simulink model "ZSM_TeslaModelS_statKreisfahrt"  (R2020b)
settings: Solver=FixedStepDiscrete  StartTime=0.0  StopTime=simtime  FixedStep=stepsize  RelTol=1e-3
undefined symbols (not defined in the file): activate_stop, activate_stop_vmax, ay_stop, ayObs, ayStiff, Bat_param, deltav_ist, DiscIntNeverNeededParam, EG_wunsch, magnitude, mu_road_LF, mu_road_LR, mu_road_RF, mu_road_RR, par_ASR, par_MDT, par_TIR, par_VEH, select_delta_h, select_M_wheel, stepsize, t, temp_betriebsstrategie, temperature_LTrange, track_left, track_right
libraries: Library_ASK x36, simulink x16, pid_lib x2, dspstat3 x2, Library_Betriebsstrategie x2, vehicle_model x2, pacejka_trans x1
(part 7 of 7)

== matlab function ZSM_TeslaModelS_statKreisfahrt/Vehicle/Betriebsstrategie/Momentenverteilung_und_Schaltstrategie1/Radmomentenaufteilung (Standardfahrmanöver)/Schaltstrategie/Schaltlogik ==
  data: delta_n_LF input; delta_n_RF input; delta_n_LR input; delta_n_RR input; delta_n_F input; delta_n_R input; delta_m_LF input; delta_m_RF input; delta_m_LR input; delta_m_RR input; delta_m_F input; delta_m_R input; idx_LF_eff input; idx_RF_eff input; idx_LR_eff input; idx_RR_eff input; idx_F_eff input; idx_R_eff input; i_LF output; i_RF output; i_LR output; i_RR output; i_F output; iv_LF input; iv_RF input; iv_LR input; iv_RR input; iv_F input; iv_R input; i_R output; idx_LF output; idx_RF output; idx_LR output; idx_RR output; idx_F output; idx_R output; idx_LF_alt input; idx_RF_alt input; idx_LR_alt input; idx_RR_alt input; idx_F_alt input; idx_R_alt input
function [i_LF, i_RF, i_LR, i_RR, i_F, i_R, idx_LF, idx_RF, idx_LR, idx_RR, idx_F, idx_R] = fcn(delta_n_LF, delta_n_RF, delta_n_LR, delta_n_RR, delta_n_F, delta_n_R, delta_m_LF, delta_m_RF, delta_m_LR, delta_m_RR, delta_m_F, delta_m_R, idx_LF_eff, idx_RF_eff, idx_LR_eff, idx_RR_eff, idx_F_eff, idx_R_eff, iv_LF, iv_RF, iv_LR, iv_RR, iv_F, iv_R, idx_LF_alt, idx_RF_alt, idx_LR_alt, idx_RR_alt, idx_F_alt, idx_R_alt)

%% Anzahl der möglichen Gänge
[A,max_LF]=size(iv_LF);
[A,max_RF]=size(iv_RF);
[A,max_LR]=size(iv_LR);
[A,max_RR]=size(iv_RR);
[A,max_F]=size(iv_F);
[A,max_R]=size(iv_R);

flag_LF=0;
flag_RF=0;
flag_LR=0;
flag_RR=0;
flag_F=0;
flag_R=0;


%% LF
idx_LF=idx_LF_alt;

if delta_n_LF<100 && idx_LF_alt<max_LF
    idx_LF=idx_LF_alt+1;
    flag_LF=1;
end

% if delta_m_LF<1 && idx_LF_alt>1 && flag_LF==0
%     idx_LF=idx_LF_alt-1;
%     flag_LF=1;
% end
    
if flag_LF==0
    idx_LF=idx_LF_eff;
end

i_LF=iv_LF(idx_LF);

%% RF
idx_RF=idx_RF_alt;

if delta_n_RF<100 && idx_RF_alt<max_RF
    idx_RF=idx_RF_alt+1;
    flag_RF=1;
end

% if delta_m_RF<1 && idx_RF_alt>1 && flag_RF==0
%     idx_RF=idx_RF_alt-1;
%     flag_RF=1;
% end
    
if flag_RF==0
    idx_RF=idx_RF_eff;
end

i_RF=iv_RF(idx_RF);

%% LR
idx_LR=idx_LR_alt;

if delta_n_LR<100 && idx_LR_alt<max_LR
    idx_LR=idx_LR_alt+1;
    flag_LR=1;
end

% if delta_m_LR<1 && idx_LR_alt>1 && flag_LR==0
%     idx_LR=idx_LR_alt-1;
%     flag_LR=1;
% end
    
if flag_LR==0
    idx_LR=idx_LR_eff;
end

i_LR=iv_LR(idx_LR);

%% RR
idx_RR=idx_RR_alt;

if delta_n_RR<100 && idx_RR_alt<max_RR
    idx_RR=idx_RR_alt+1;
    flag_RR=1;
end

% if delta_m_RR<1 && idx_RR_alt>1 && flag_RR==0
%     idx_RR=idx_RR_alt-1;
%     flag_RR=1;
% end
    
if flag_RR==0
    idx_RR=idx_RR_eff;
end

i_RR=iv_RR(idx_RR);

%% F
idx_F=idx_F_alt;

if delta_n_F<100 && idx_F_alt<max_F
    idx_F=idx_F_alt+1;
    flag_F=1;
end

% if delta_m_F<1 && idx_F_alt>1 && flag_F==0
%     idx_F=idx_F_alt-1;
%     flag_F=1;
% end
    
if flag_F==0
    idx_F=idx_F_eff;
end

i_F=iv_F(idx_F);

%% R
idx_R=idx_R_alt;

if delta_n_R<100 && idx_R_alt<max_R
    idx_R=idx_R_alt+1;
    flag_R=1;
end

% if delta_m_R<1 && idx_R_alt>1 && flag_R==0
%     idx_R=idx_R_alt-1;
%     flag_R=1;
% end
    
if flag_R==0
    idx_R=idx_R_eff;
end

i_R=iv_R(idx_R);

== matlab function ZSM_TeslaModelS_statKreisfahrt/Vehicle/Betriebsstrategie/Momentenverteilung_und_Schaltstrategie1/Radmomentenaufteilung (Standardfahrmanöver)/Schaltstrategie/effizientester Gang ==
  data: eta_LF input; eta_RF input; eta_LR input; eta_RR input; eta_F input; eta_R input; idx_LF_eff output; idx_RF_eff output; idx_LR_eff output; idx_RR_eff output; idx_F_eff output; idx_R_eff output; eta_trans_F input; eta_trans_R input
function [idx_LF_eff, idx_RF_eff, idx_LR_eff, idx_RR_eff, idx_F_eff, idx_R_eff] = fcn(eta_LF, eta_RF, eta_LR, eta_RR, eta_F, eta_R, eta_trans_F, eta_trans_R)

%% effizientester Gang Achszentraler Aufbau
[A,B]=max(eta_F .* eta_trans_F);
idx_F_eff=B;

[A,B]=max(eta_R .* eta_trans_R);
idx_R_eff=B;

%% effizientester Gang Radindividueller Aufbau
[A,B]=max(eta_LF .* eta_trans_F);
idx_LF_eff=B;

[A,B]=max(eta_RF .* eta_trans_F);
idx_RF_eff=B;

[A,B]=max(eta_LR .* eta_trans_R);
idx_LR_eff=B;

[A,B]=max(eta_RR .* eta_trans_R);
idx_RR_eff=B;

== matlab function ZSM_TeslaModelS_statKreisfahrt/Vehicle/Betriebsstrategie/Momentenverteilung_und_Schaltstrategie1/Radmomentenaufteilung (Standardfahrmanöver)/Schaltstrategie/n und Motordrehmoment als Vektor (wegen ALLEN Übersetzungen) ==
  data: omega_LF input; n_LF output; m_LF output; omega_RF input; omega_LR input; omega_RR input; M_LF input; M_RF input; M_LR input; M_RR input; i_LF input; i_RF input; i_LR input; i_RR input; i_F input; i_R input; n_RF output; m_RF output; n_LR output; m_LR output; n_RR output; m_RR output; n_F output; m_F output; n_R output; m_R output
function [n_LF,m_LF, n_RF,m_RF, n_LR,m_LR, n_RR,m_RR, n_F,m_F, n_R,m_R] = fcn(omega_LF, omega_RF, omega_LR, omega_RR, M_LF, M_RF, M_LR, M_RR, i_LF, i_RF, i_LR, i_RR, i_F, i_R)

%% Drehzahlen und Momente als Vektoren
% Die Menge an möglichen Übersetzungen liegt als Vektor vor.
% Durch Vektoropertaionen werden Drehzahlen und Momente ebenfalls als
% Vektoren dargestellt. Diese werden im Wirkungsgradkennfeld zu einem
% Vektor an Wirkungsgraden. Von diesen wird der beste ausgewählt.

%% Raddrehzahlen Achszentraler Aufbau
n_F = (omega_LF+omega_RF)*0.5.*i_F;
n_R = (omega_LR+omega_RR)*0.5.*i_R;

%% Raddrehzahlen Radindividueller Aufbau
n_LF = omega_LF.*i_LF;
n_RF = omega_RF.*i_RF;
n_LR = omega_LR.*i_LR;
n_RR = omega_RR.*i_RR;

%% Motormoment Achszentraler Aufbau
m_F=(M_LF+M_RF)./i_F;
m_R=(M_LR+M_RR)./i_R;

%% Motormoment Radindividueller Aufbau
m_LF=M_LF./i_LF;
m_RF=M_RF./i_RF;
m_LR=M_LR./i_LR;
m_RR=M_RR./i_RR;

== matlab function ZSM_TeslaModelS_statKreisfahrt/Vehicle/Betriebsstrategie/Momentenverteilung_und_Schaltstrategie1/Radmomentenaufteilung (Standardfahrmanöver)/Schaltstrategie/omega zu n ==
  data: omega_LF input; n_LF output; omega_RF input; omega_LR input; omega_RR input; i_LF input; i_RF input; i_LR input; i_RR input; i_F input; i_R input; n_RF output; n_LR output; n_RR output; n_F output; n_R output
function [n_LF, n_RF, n_LR, n_RR, n_F, n_R] = fcn(omega_LF, omega_RF, omega_LR, omega_RR, i_LF, i_RF, i_LR, i_RR, i_F, i_R)

%% Raddrehzahlen Achszentraler Aufbau
n_F = (omega_LF+omega_RF)*0.5*i_F;
n_R = (omega_LR+omega_RR)*0.5*i_R;

%% Raddrehzahlen Radindividueller Aufbau
n_LF = omega_LF*i_LF;
n_RF = omega_RF*i_RF;
n_LR = omega_LR*i_LR;
n_RR = omega_RR*i_RR;

== matlab function ZSM_TeslaModelS_statKreisfahrt/Driver/Splines/Kennwerte ==
  data: psi_old input; psi_spline output; time input; a1 input; a0 input; v2 input; v1 input; v0 input; p3 input; p2 input; p1 input; p0 input; psi_real input; spl_a_glob output; spl_v_glob output; spl_p_glob output; spl_a_veh output; spl_v_veh output; p_err_long output; p_ist input; p_err_lat output
function [ psi_spline, spl_a_glob, spl_v_glob, spl_p_glob, spl_a_veh, spl_v_veh, p_err_long, p_err_lat]   = Kennwerte(psi_old, time, a1, a0, v2, v1, v0, p3, p2, p1, p0, psi_real, p_ist) 
%Splinekoeffizienten im Abstand von 0.01 s, deshalb wird Zeit mit 100 
%mulitpliziert,um alle 0.01 s auf nächsten Spline-Koeffizienten zuzugreifen
time = time * 100;
%t wird angelegt, damit extrapoliert werden kann, wenn die Zeit über die
%vorgesehene Zeit im Struct hinausreicht
t = time;
if time > length(a0)-2
    time = length(a0)-2;
end

si = int16(floor(time)+1); %Spline Index, Auswahl des Richtigen Splines 
ov = t-floor(time); %Overshoot, Zeit nach dem Beginn des Spline

%%Berechnung der Beschleunigung a, Geschwindigkeit v und Position p in globalen Koordianten
spl_a_glob =  a1(:,si).*(ov)   +a0(:,si);
spl_v_glob =  v2(:,si).*(ov).^2+v1(:,si).*(ov)   +v0(:,si);
spl_p_glob =  p3(:,si).*(ov).^3+p2(:,si).*(ov).^2+p1(:,si).*(ov)+p0(:,si);

%%Verhindert Springen des Gierwinkels bei niedrigen Geschwindigkeiten
if spl_v_glob(1) < 1e-5 && spl_v_glob(2) < 1e-5
     psi_spline = psi_old;
else
     psi_spline = atan2(spl_v_glob(2),spl_v_glob(1)); %Gierwinkel soll
end

psi = psi_spline; %Optional kann die tatsächliche Fahrzeugausrichtung verwendet werden
tm  = [cos(psi) sin(psi); -sin(psi) cos(psi)]; %Transformations-Matrix

spl_a_veh = tm * spl_a_glob; %Beschleunigung soll in Fahrzeugsollkoordinaten
spl_v_veh = tm * spl_v_glob; %Geschwindigkeit soll in Fahrzeugsollkoordinaten


p_veh = tm * (p_ist - spl_p_glob);
p_err_long = p_veh(1); %Lateraler Fehler in Fahrzeugsollkoordinaten
p_err_lat = p_veh(2); %Longitudinaler in Fahrzeugsollkoordinaten

end

== matlab function ZSM_TeslaModelS_statKreisfahrt/Vehicle/Antriebsstrang und Radmomentenverteilung/Batterie/MATLAB Function2 ==
  data: u input; y output
function y = fcn(u)
%Transponieren der Leistung -> für das Batteriemodell

y=reshape(u,[1,1,[]]);


end

== matlab function ZSM_TeslaModelS_statKreisfahrt/Vehicle/Betriebsstrategie/Momentenverteilung_und_Schaltstrategie1/Radmomentenaufteilung (Effizienz)/Momentenrückführung und Motormomentberechnung/Getriebewirkungsgradberechnung Vorderachse/MATLAB Function ==
  data: M_out input; M_in output; M_max input
function M_in = fcn(M_out, M_max)
M_in = 3/680 *((sqrt(M_max) * sqrt(27*M_max + 27200*M_out))/sqrt(3) - 3 * M_max)
